simulink model "dac_driver"  (R2012b)
settings: Solver=ode45  StartTime=0.0  StopTime=10.0  RelTol=1e-3
undefined symbols (not defined in the file or in its folder): gcbh, xlBlockLoadCallback, xlGetNormalizedPeriod
libraries: xbsIndex_r4 x54, xbsEDKLib_r4 x1
(part 1 of 2)
settings Model: Creator=rcagley  LastModifiedBy=rcagley
settings DataIOCC: SignalLoggingSaveFormat=ModelDataLogs
settings DebuggingCC: FcnCallInpInsideContextMsg=EnableAllAsWarning

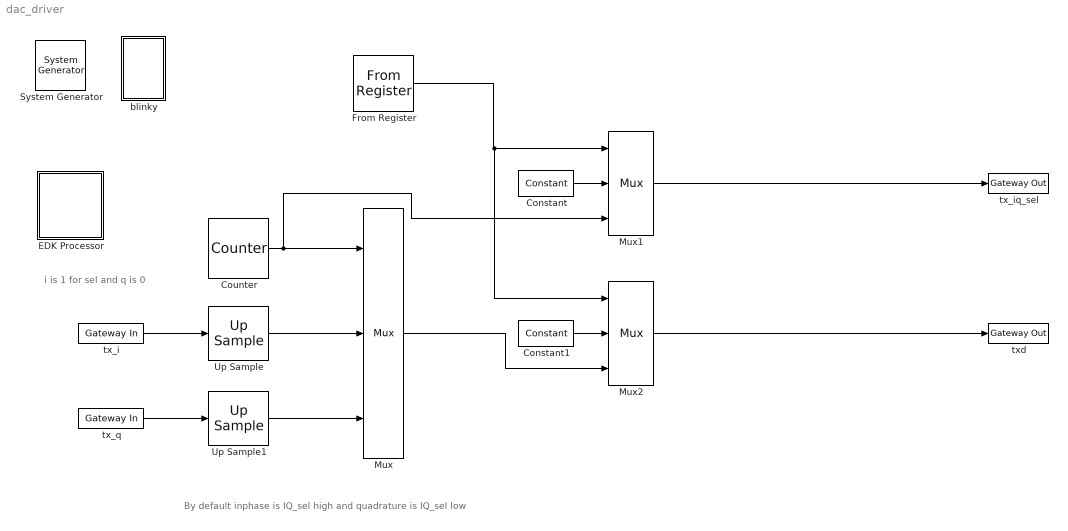
== system dac_driver ==
  note: i is 1 for sel and q is 0
  note: By default inphase is IQ_sel high and quadrature is IQ_sel low
  " System Generator" : xbsIndex_r4/ System Generator  Tag=genX  xilinxfamily=zynq  part=xc7z020  speed=-1  package=clg484  synthesis_tool=XST  clock_wrapper=Clock Enables  directory=./netlist  proj_type=Project Navigator  Synth_file=XST Defaults  Impl_file=ISE Defaults  testbench=off  simulink_period=1  sysclk_period=10  dcm_input_clock_period=10  incr_netlist=off  trim_vbits=Everywhere in SubSystem  dbl_ovrd=According to Block Masks  core_generation=According to Block Masks  run_coregen=off  deprecated_control=off  eval_field=0  block_type=sysgen
  Constant : xbsIndex_r4/Constant  const=0  gui_display_data_type=Fixed-point  arith_type=Unsigned  n_bits=1  bin_pt=0  preci_type=Single  exp_width=8  frac_width=24  explicit_period=on  period=1  equ=P=C  opselect=C  inp2=PCIN>>17  opr=+  inp1=P  carry=CIN  dbl_ovrd=off  block_type=constant
  Constant1 : xbsIndex_r4/Constant  const=0  gui_display_data_type=Fixed-point  arith_type=Signed (2's comp)  n_bits=12  bin_pt=0  preci_type=Single  exp_width=8  frac_width=24  explicit_period=on  period=1  equ=P=C  opselect=C  inp2=PCIN>>17  opr=+  inp1=P  carry=CIN  dbl_ovrd=off  block_type=constant
  Counter : xbsIndex_r4/Counter  cnt_type=Free Running  cnt_to=Inf  operation=Up  start_count=0  cnt_by_val=1  arith_type=Unsigned  n_bits=1  bin_pt=0  load_pin=off  rst=off  en=off  explicit_period=on  period=1  dbl_ovrd=off  use_behavioral_HDL=off  implementation=Fabric  block_type=counter
  EDK Processor : Subsystem  LoadFcn=xlBlockLoadCallback(gcbh);  mask(Xilinx EDK Processor Block){mode=EDK pcore generation, xmp=, MemVisToProc=<qt bgcolor="#FFFFFF"><div><img src="C:/Xilinx/14.2/ISE_DS/ISE/sysgen/data/images/registerplus.gif"> &lt;&lt;dac_en&gt;&gt;<br></div></qt>, AvailableMemories=<empty>, portInterfaceTable={'exposed'=>[],'portdir'=>[],'portname'=>[],'shortname'=>[]}, bus_type_sgadvanced=, bus_type=AXI, baseaddr=0x80000000, baseaddr_lock_sgadvanced=, baseaddr_lock=off, dual_clock_sgadvanced=, dual_clock=on, reg_readback_sgadvanced=, reg_readback=off, ucf_file=, inheritDeviceType_sgadvanced=, inheritDeviceType=off, elf_file=, codebug_sgadvanced=, codebug=on, clock_name=plb, internalPortList={}, resetPolarity=0, memxtable={'mladdr'=>[0.00000000000000000],'mlist'=>['dac_driver/From Register'],'mlname'=>['\'dac_en\''],'mlstate'=>[0.00000000000000000]}, procinfo={}, memmapdirty=off, blockname=, xpsintstyle=default, has_advanced_control=0, sggui_pos=-1,-1,-1,-1, block_type=edkprocessor, block_version=2.7, sg_icon_stat=62,64,-1,-1,white,blue,0,07734,right,,[ ],[ ], sg_mask_display=|, sg_list_contents={'table'=>{'AvailableMemories'=>'popup(<empty>)'}}, sg_blockgui_xml=}
      mask sg_mask_display=|
      | fprintf('','COMMENT: begin icon graphics');
      | patch([0 62 62 0 0 ],[0 0 64 64 0 ],[0.77 0.82 0.91 ]);
      | plot([0 62 62 0 0 ],[0 0 64 64 0 ]);
      | patch([13.2 24.76 32.76 40.76 48.76 32.76 21.2 13.2 ],[40.88 40.88 48.88 40.88 48.88 48.88 48.88 40.88 ],[1 1 1 ]);
      | patch([21.2 32.76 24.76 13.2 21.2 ],[32.88 32.88 40.88 40.88 32.88 ],[0.931 0.946 0.973 ]);
      | patch([13.2 24.76 32.76 21.2 13.2 ],[24.88 24.88 32.88 32.88 24.88 ],[1 1 1 ]);
      | patch([21.2 48.76 40.76 32.76 24.76 13.2 21.2 ],[16.88 16.88 24.88 16.88 24.88 24.88 16.88 ],[0.931 0.946 0.973 ]);
      | fprintf('','COMMENT: end icon graphics');
      | fprintf('','COMMENT: begin icon text');
      | fprintf('','COMMENT: end icon text');
      mask prompts: mode "Configure Processor for"; xmp "XPS Project"; MemVisToProc ""; AvailableMemories "Available Memories"; portInterfaceTable ""; bus_type_sgadvanced ""; bus_type "Bus Type"; baseaddr "Base Address"; baseaddr_lock_sgadvanced ""; baseaddr_lock "Lock"; dual_clock_sgadvanced ""; dual_clock "Dual Clocks"; reg_readback_sgadvanced ""; reg_readback "Register Read-Back"; ucf_file "Constraint File"; inheritDeviceType_sgadvanced ""; inheritDeviceType "Inherit Device Type"; elf_file "Initial Program"; codebug_sgadvanced ""; codebug "Enable Co-Debug with Xilinx SDK (Beta)"; clock_name ""; internalPortList ""; resetPolarity ""; memxtable ""; procinfo ""; memmapdirty ""; blockname ""; xpsintstyle ""; has_advanced_control ""; sggui_pos ""; block_type ""; block_version ""; sg_icon_stat ""; sg_mask_display ""; sg_list_contents ""; sg_blockgui_xml ""
      mask help: Xilinx EDK Processor
      mask init:
      | try
      |   tmp_gcb = gcb;
      |   tmp_gcbh = gcbh;
      |   if (strcmp('SysGenIndex',get_param(bdroot(tmp_gcbh),'tag')) && ~isempty(regexp(bdroot(tmp_gcb), '^xbs', 'once')))
      |     return;
      |   end;
      |   xlMungeMaskParams;
      | 
      |   block_type='edkprocessor';
      | 
      |   serialized_declarations = '{''block_type''=>''String''}';
      |   xledkprocessor_init();
      |   ptable_ = xlblockprep(get_param(tmp_gcb, 'MaskWSVariables'));
      |   try
      |     xlBlockMoveCallback(tmp_gcbh);
      |   catch 
      |      clear global xl_updateicon_recursion_guard;
      |   end;
      | catch
      |   global dbgsysgen;
      |   if(~isempty(dbgsysgen) && dbgsysgen)
      |     e = regexprep(lasterr, '\n', '\nError: ');
      |     disp(['Error: While running MaskInit code on block ' tmp_gcb ': ' e]);
      |     error(e);
      |   end
      | end
      settings: CopyFcn=xlProcBlockCopyCallback(gcbh);xlBlockMoveCallback(gcbh);  DeleteFcn=xlDestroyGui(gcbh);  ModelCloseFcn=xlDestroyGui(gcbh);  PreSaveFcn=xlBlockPreSaveCallback(gcbh);  PostSaveFcn=xlBlockPostSaveCallback(gcbh);  DestroyFcn=xlDestroyGui(gcbh);  OpenFcn=bh=gcbh;xlProcBlockCallbacks('populatesharedmemorylistbox',bh);xlOpenGui(bh, 'edkprocessor_gui.xml', @xlProcBlockEnablement, @xlProcBlockAction);  CloseFcn=xlDestroyGui(gcbh);  MoveFcn=xlBlockMoveCallback(gcbh);
      mask Help: eval('');xlDoc('-book','sysgen','-topic','EDK_Processor');
      mask TypeOptions mode: EDK pcore generation | HDL netlisting
      mask TypeOptions bus_type: AXI | PLB
      mask Display:
      | fprintf('','COMMENT: begin icon graphics');
      | patch([0 62 62 0 0 ],[0 0 64 64 0 ],[0.77 0.82 0.91 ]);
      | plot([0 62 62 0 0 ],[0 0 64 64 0 ]);
      | patch([13.2 24.76 32.76 40.76 48.76 32.76 21.2 13.2 ],[40.88 40.88 48.88 40.88 48.88 48.88 48.88 40.88 ],[1 1 1 ]);
      | patch([21.2 32.76 24.76 13.2 21.2 ],[32.88 32.88 40.88 40.88 32.88 ],[0.931 0.946 0.973 ]);
      | patch([13.2 24.76 32.76 21.2 13.2 ],[24.88 24.88 32.88 32.88 24.88 ],[1 1 1 ]);
      | patch([21.2 48.76 40.76 32.76 24.76 13.2 21.2 ],[16.88 16.88 24.88 16.88 24.88 24.88 16.88 ],[0.931 0.946 0.973 ]);
      | fprintf('','COMMENT: end icon graphics');
      | fprintf('','COMMENT: begin icon text');
      | disp('');
      | 
      | fprintf('','COMMENT: end icon text');
  From Register : xbsIndex_r4/From Register  shared_memory_name='dac_en'  init=0  period=1  ownership=Locally owned and initialized  gui_display_data_type=Fixed-point  arith_type=Unsigned  n_bits=1  bin_pt=0  preci_type=Single  dbl_ovrd=off  block_type=fromreg
      settings: AttributesFormatString=<< %<shared_memory_name> >>  infoedit="Register block that reads data to a shared memory register.  Delay of one sample period."
  Mux : xbsIndex_r4/Mux  inputs=2  en=off  latency=0  precision=Full  arith_type=Unsigned  n_bits=16  bin_pt=14  quantization=Truncate  overflow=Wrap  dbl_ovrd=off  block_type=mux
  Mux1 : xbsIndex_r4/Mux  inputs=2  en=off  latency=0  precision=Full  arith_type=Unsigned  n_bits=16  bin_pt=14  quantization=Truncate  overflow=Wrap  dbl_ovrd=off  block_type=mux
  Mux2 : xbsIndex_r4/Mux  inputs=2  en=off  latency=0  precision=Full  arith_type=Unsigned  n_bits=16  bin_pt=14  quantization=Truncate  overflow=Wrap  dbl_ovrd=off  block_type=mux
  Up Sample : xbsIndex_r4/Up Sample  sample_ratio=2  copy_samples=on  en=off  latency=0  dbl_ovrd=off  block_type=usamp
  Up Sample1 : xbsIndex_r4/Up Sample  sample_ratio=2  copy_samples=on  en=off  latency=0  dbl_ovrd=off  block_type=usamp
  blinky : Subsystem
  tx_i : xbsIndex_r4/Gateway In  gui_display_data_type=Fixed-point  arith_type="Signed  (2's comp)"  n_bits=12  bin_pt=0  preci_type=Single  exp_width=8  frac_width=24  quantization="Round  (unbiased: +/- Inf)"  overflow=Saturate  period=2  dbl_ovrd=off  timing_constraint=None  locs_specified=off  LOCs={}  UseAsADC=off  ADCChannel='1'  inherit_from_input=off  hdl_port=on  block_type=gatewayin
  tx_iq_sel : xbsIndex_r4/Gateway Out  inherit_from_input=off  hdl_port=on  timing_constraint=None  locs_specified=off  LOCs={}  UseAsDAC=off  DACChannel='1'  block_type=gatewayout
  tx_q : xbsIndex_r4/Gateway In  gui_display_data_type=Fixed-point  arith_type="Signed  (2's comp)"  n_bits=12  bin_pt=0  preci_type=Single  exp_width=8  frac_width=24  quantization="Round  (unbiased: +/- Inf)"  overflow=Saturate  period=2  dbl_ovrd=off  timing_constraint=None  locs_specified=off  LOCs={}  UseAsADC=off  ADCChannel='1'  inherit_from_input=off  hdl_port=on  block_type=gatewayin
  txd : xbsIndex_r4/Gateway Out  inherit_from_input=off  hdl_port=on  timing_constraint=None  locs_specified=off  LOCs={}  UseAsDAC=off  DACChannel='1'  block_type=gatewayout
  wires:
  Up Sample/1 -> Mux/2
  Up Sample1/1 -> Mux/3
  Counter/1 -> Mux/1, Mux1/3
  Mux2/1 -> txd/1
  Mux1/1 -> tx_iq_sel/1
  Mux/1 -> Mux2/3
  From Register/1 -> Mux2/1, Mux1/1
  Constant/1 -> Mux1/2
  Constant1/1 -> Mux2/2
  tx_i/1 -> Up Sample/1
  tx_q/1 -> Up Sample1/1

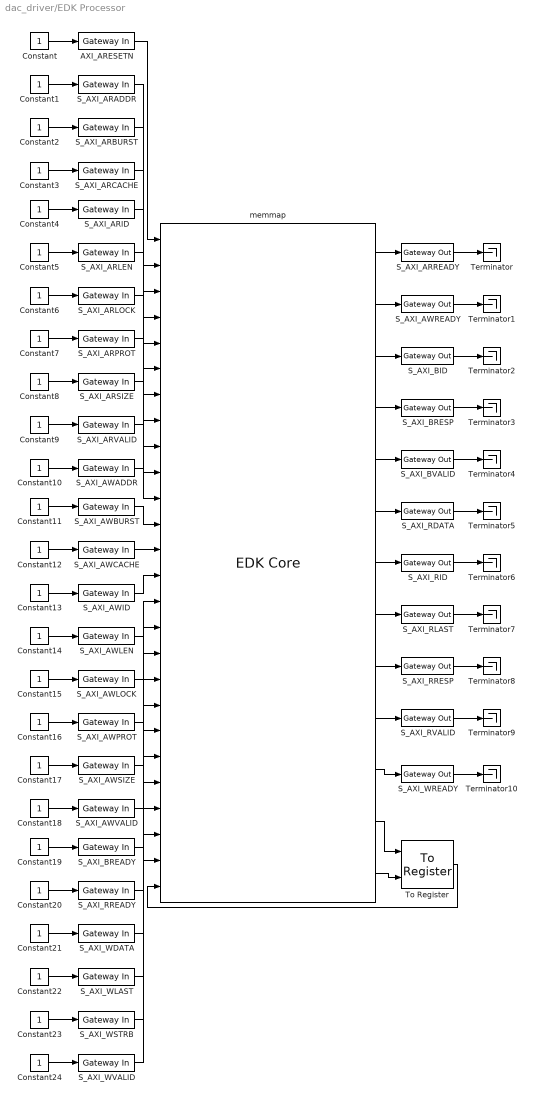
== system dac_driver/EDK Processor ==
  AXI_ARESETN : xbsIndex_r4/Gateway In  gui_display_data_type=Fixed-point  arith_type=Boolean  n_bits=16  bin_pt=14  preci_type=Single  exp_width=8  frac_width=24  quantization="Round  (unbiased: +/- Inf)"  overflow=Saturate  period=xlGetNormalizedPeriod()  dbl_ovrd=off  timing_constraint=None  locs_specified=off  LOCs={}  UseAsADC=off  ADCChannel='1'  inherit_from_input=off  hdl_port=on  block_type=gatewayin
  Constant{,1..24} (25 alike) : Constant
  S_AXI_ARADDR : xbsIndex_r4/Gateway In  gui_display_data_type=Fixed-point  arith_type=Unsigned  n_bits=32  bin_pt=0  preci_type=Single  exp_width=8  frac_width=24  quantization="Round  (unbiased: +/- Inf)"  overflow=Saturate  period=xlGetNormalizedPeriod()  dbl_ovrd=off  timing_constraint=None  locs_specified=off  LOCs={}  UseAsADC=off  ADCChannel='1'  inherit_from_input=off  hdl_port=on  block_type=gatewayin
  S_AXI_ARBURST : xbsIndex_r4/Gateway In  gui_display_data_type=Fixed-point  arith_type=Unsigned  n_bits=2  bin_pt=0  preci_type=Single  exp_width=8  frac_width=24  quantization="Round  (unbiased: +/- Inf)"  overflow=Saturate  period=xlGetNormalizedPeriod()  dbl_ovrd=off  timing_constraint=None  locs_specified=off  LOCs={}  UseAsADC=off  ADCChannel='1'  inherit_from_input=off  hdl_port=on  block_type=gatewayin
  S_AXI_ARCACHE : xbsIndex_r4/Gateway In  gui_display_data_type=Fixed-point  arith_type=Unsigned  n_bits=4  bin_pt=0  preci_type=Single  exp_width=8  frac_width=24  quantization="Round  (unbiased: +/- Inf)"  overflow=Saturate  period=xlGetNormalizedPeriod()  dbl_ovrd=off  timing_constraint=None  locs_specified=off  LOCs={}  UseAsADC=off  ADCChannel='1'  inherit_from_input=off  hdl_port=on  block_type=gatewayin
  S_AXI_ARID : xbsIndex_r4/Gateway In  gui_display_data_type=Fixed-point  arith_type=Unsigned  n_bits=8  bin_pt=0  preci_type=Single  exp_width=8  frac_width=24  quantization="Round  (unbiased: +/- Inf)"  overflow=Saturate  period=xlGetNormalizedPeriod()  dbl_ovrd=off  timing_constraint=None  locs_specified=off  LOCs={}  UseAsADC=off  ADCChannel='1'  inherit_from_input=off  hdl_port=on  block_type=gatewayin
  S_AXI_ARLEN : xbsIndex_r4/Gateway In  gui_display_data_type=Fixed-point  arith_type=Unsigned  n_bits=8  bin_pt=0  preci_type=Single  exp_width=8  frac_width=24  quantization="Round  (unbiased: +/- Inf)"  overflow=Saturate  period=xlGetNormalizedPeriod()  dbl_ovrd=off  timing_constraint=None  locs_specified=off  LOCs={}  UseAsADC=off  ADCChannel='1'  inherit_from_input=off  hdl_port=on  block_type=gatewayin
  S_AXI_ARLOCK : xbsIndex_r4/Gateway In  gui_display_data_type=Fixed-point  arith_type=Unsigned  n_bits=2  bin_pt=0  preci_type=Single  exp_width=8  frac_width=24  quantization="Round  (unbiased: +/- Inf)"  overflow=Saturate  period=xlGetNormalizedPeriod()  dbl_ovrd=off  timing_constraint=None  locs_specified=off  LOCs={}  UseAsADC=off  ADCChannel='1'  inherit_from_input=off  hdl_port=on  block_type=gatewayin
  S_AXI_ARPROT : xbsIndex_r4/Gateway In  gui_display_data_type=Fixed-point  arith_type=Unsigned  n_bits=3  bin_pt=0  preci_type=Single  exp_width=8  frac_width=24  quantization="Round  (unbiased: +/- Inf)"  overflow=Saturate  period=xlGetNormalizedPeriod()  dbl_ovrd=off  timing_constraint=None  locs_specified=off  LOCs={}  UseAsADC=off  ADCChannel='1'  inherit_from_input=off  hdl_port=on  block_type=gatewayin
  S_AXI_ARREADY : xbsIndex_r4/Gateway Out  inherit_from_input=off  hdl_port=on  timing_constraint=None  locs_specified=off  LOCs={}  UseAsDAC=off  DACChannel='1'  block_type=gatewayout
  S_AXI_ARSIZE : xbsIndex_r4/Gateway In  gui_display_data_type=Fixed-point  arith_type=Unsigned  n_bits=3  bin_pt=0  preci_type=Single  exp_width=8  frac_width=24  quantization="Round  (unbiased: +/- Inf)"  overflow=Saturate  period=xlGetNormalizedPeriod()  dbl_ovrd=off  timing_constraint=None  locs_specified=off  LOCs={}  UseAsADC=off  ADCChannel='1'  inherit_from_input=off  hdl_port=on  block_type=gatewayin
  S_AXI_ARVALID : xbsIndex_r4/Gateway In  gui_display_data_type=Fixed-point  arith_type=Boolean  n_bits=16  bin_pt=14  preci_type=Single  exp_width=8  frac_width=24  quantization="Round  (unbiased: +/- Inf)"  overflow=Saturate  period=xlGetNormalizedPeriod()  dbl_ovrd=off  timing_constraint=None  locs_specified=off  LOCs={}  UseAsADC=off  ADCChannel='1'  inherit_from_input=off  hdl_port=on  block_type=gatewayin
  S_AXI_AWADDR : xbsIndex_r4/Gateway In  gui_display_data_type=Fixed-point  arith_type=Unsigned  n_bits=32  bin_pt=0  preci_type=Single  exp_width=8  frac_width=24  quantization="Round  (unbiased: +/- Inf)"  overflow=Saturate  period=xlGetNormalizedPeriod()  dbl_ovrd=off  timing_constraint=None  locs_specified=off  LOCs={}  UseAsADC=off  ADCChannel='1'  inherit_from_input=off  hdl_port=on  block_type=gatewayin
  S_AXI_AWBURST : xbsIndex_r4/Gateway In  gui_display_data_type=Fixed-point  arith_type=Unsigned  n_bits=2  bin_pt=0  preci_type=Single  exp_width=8  frac_width=24  quantization="Round  (unbiased: +/- Inf)"  overflow=Saturate  period=xlGetNormalizedPeriod()  dbl_ovrd=off  timing_constraint=None  locs_specified=off  LOCs={}  UseAsADC=off  ADCChannel='1'  inherit_from_input=off  hdl_port=on  block_type=gatewayin
  S_AXI_AWCACHE : xbsIndex_r4/Gateway In  gui_display_data_type=Fixed-point  arith_type=Unsigned  n_bits=4  bin_pt=0  preci_type=Single  exp_width=8  frac_width=24  quantization="Round  (unbiased: +/- Inf)"  overflow=Saturate  period=xlGetNormalizedPeriod()  dbl_ovrd=off  timing_constraint=None  locs_specified=off  LOCs={}  UseAsADC=off  ADCChannel='1'  inherit_from_input=off  hdl_port=on  block_type=gatewayin
  S_AXI_AWID : xbsIndex_r4/Gateway In  gui_display_data_type=Fixed-point  arith_type=Unsigned  n_bits=8  bin_pt=0  preci_type=Single  exp_width=8  frac_width=24  quantization="Round  (unbiased: +/- Inf)"  overflow=Saturate  period=xlGetNormalizedPeriod()  dbl_ovrd=off  timing_constraint=None  locs_specified=off  LOCs={}  UseAsADC=off  ADCChannel='1'  inherit_from_input=off  hdl_port=on  block_type=gatewayin
  S_AXI_AWLEN : xbsIndex_r4/Gateway In  gui_display_data_type=Fixed-point  arith_type=Unsigned  n_bits=8  bin_pt=0  preci_type=Single  exp_width=8  frac_width=24  quantization="Round  (unbiased: +/- Inf)"  overflow=Saturate  period=xlGetNormalizedPeriod()  dbl_ovrd=off  timing_constraint=None  locs_specified=off  LOCs={}  UseAsADC=off  ADCChannel='1'  inherit_from_input=off  hdl_port=on  block_type=gatewayin
  S_AXI_AWLOCK : xbsIndex_r4/Gateway In  gui_display_data_type=Fixed-point  arith_type=Unsigned  n_bits=2  bin_pt=0  preci_type=Single  exp_width=8  frac_width=24  quantization="Round  (unbiased: +/- Inf)"  overflow=Saturate  period=xlGetNormalizedPeriod()  dbl_ovrd=off  timing_constraint=None  locs_specified=off  LOCs={}  UseAsADC=off  ADCChannel='1'  inherit_from_input=off  hdl_port=on  block_type=gatewayin
  S_AXI_AWPROT : xbsIndex_r4/Gateway In  gui_display_data_type=Fixed-point  arith_type=Unsigned  n_bits=3  bin_pt=0  preci_type=Single  exp_width=8  frac_width=24  quantization="Round  (unbiased: +/- Inf)"  overflow=Saturate  period=xlGetNormalizedPeriod()  dbl_ovrd=off  timing_constraint=None  locs_specified=off  LOCs={}  UseAsADC=off  ADCChannel='1'  inherit_from_input=off  hdl_port=on  block_type=gatewayin
  S_AXI_AWREADY : xbsIndex_r4/Gateway Out  inherit_from_input=off  hdl_port=on  timing_constraint=None  locs_specified=off  LOCs={}  UseAsDAC=off  DACChannel='1'  block_type=gatewayout
  S_AXI_AWSIZE : xbsIndex_r4/Gateway In  gui_display_data_type=Fixed-point  arith_type=Unsigned  n_bits=3  bin_pt=0  preci_type=Single  exp_width=8  frac_width=24  quantization="Round  (unbiased: +/- Inf)"  overflow=Saturate  period=xlGetNormalizedPeriod()  dbl_ovrd=off  timing_constraint=None  locs_specified=off  LOCs={}  UseAsADC=off  ADCChannel='1'  inherit_from_input=off  hdl_port=on  block_type=gatewayin
  S_AXI_AWVALID : xbsIndex_r4/Gateway In  gui_display_data_type=Fixed-point  arith_type=Boolean  n_bits=16  bin_pt=14  preci_type=Single  exp_width=8  frac_width=24  quantization="Round  (unbiased: +/- Inf)"  overflow=Saturate  period=xlGetNormalizedPeriod()  dbl_ovrd=off  timing_constraint=None  locs_specified=off  LOCs={}  UseAsADC=off  ADCChannel='1'  inherit_from_input=off  hdl_port=on  block_type=gatewayin
  S_AXI_BID : xbsIndex_r4/Gateway Out  inherit_from_input=off  hdl_port=on  timing_constraint=None  locs_specified=off  LOCs={}  UseAsDAC=off  DACChannel='1'  block_type=gatewayout
  S_AXI_BREADY : xbsIndex_r4/Gateway In  gui_display_data_type=Fixed-point  arith_type=Boolean  n_bits=16  bin_pt=14  preci_type=Single  exp_width=8  frac_width=24  quantization="Round  (unbiased: +/- Inf)"  overflow=Saturate  period=xlGetNormalizedPeriod()  dbl_ovrd=off  timing_constraint=None  locs_specified=off  LOCs={}  UseAsADC=off  ADCChannel='1'  inherit_from_input=off  hdl_port=on  block_type=gatewayin
  S_AXI_BRESP : xbsIndex_r4/Gateway Out  inherit_from_input=off  hdl_port=on  timing_constraint=None  locs_specified=off  LOCs={}  UseAsDAC=off  DACChannel='1'  block_type=gatewayout
  S_AXI_BVALID : xbsIndex_r4/Gateway Out  inherit_from_input=off  hdl_port=on  timing_constraint=None  locs_specified=off  LOCs={}  UseAsDAC=off  DACChannel='1'  block_type=gatewayout
  S_AXI_RDATA : xbsIndex_r4/Gateway Out  inherit_from_input=off  hdl_port=on  timing_constraint=None  locs_specified=off  LOCs={}  UseAsDAC=off  DACChannel='1'  block_type=gatewayout
  S_AXI_RID : xbsIndex_r4/Gateway Out  inherit_from_input=off  hdl_port=on  timing_constraint=None  locs_specified=off  LOCs={}  UseAsDAC=off  DACChannel='1'  block_type=gatewayout
  S_AXI_RLAST : xbsIndex_r4/Gateway Out  inherit_from_input=off  hdl_port=on  timing_constraint=None  locs_specified=off  LOCs={}  UseAsDAC=off  DACChannel='1'  block_type=gatewayout
  S_AXI_RREADY : xbsIndex_r4/Gateway In  gui_display_data_type=Fixed-point  arith_type=Boolean  n_bits=16  bin_pt=14  preci_type=Single  exp_width=8  frac_width=24  quantization="Round  (unbiased: +/- Inf)"  overflow=Saturate  period=xlGetNormalizedPeriod()  dbl_ovrd=off  timing_constraint=None  locs_specified=off  LOCs={}  UseAsADC=off  ADCChannel='1'  inherit_from_input=off  hdl_port=on  block_type=gatewayin
  S_AXI_RRESP : xbsIndex_r4/Gateway Out  inherit_from_input=off  hdl_port=on  timing_constraint=None  locs_specified=off  LOCs={}  UseAsDAC=off  DACChannel='1'  block_type=gatewayout
  S_AXI_RVALID : xbsIndex_r4/Gateway Out  inherit_from_input=off  hdl_port=on  timing_constraint=None  locs_specified=off  LOCs={}  UseAsDAC=off  DACChannel='1'  block_type=gatewayout
  S_AXI_WDATA : xbsIndex_r4/Gateway In  gui_display_data_type=Fixed-point  arith_type=Unsigned  n_bits=32  bin_pt=0  preci_type=Single  exp_width=8  frac_width=24  quantization="Round  (unbiased: +/- Inf)"  overflow=Saturate  period=xlGetNormalizedPeriod()  dbl_ovrd=off  timing_constraint=None  locs_specified=off  LOCs={}  UseAsADC=off  ADCChannel='1'  inherit_from_input=off  hdl_port=on  block_type=gatewayin
  S_AXI_WLAST : xbsIndex_r4/Gateway In  gui_display_data_type=Fixed-point  arith_type=Boolean  n_bits=16  bin_pt=14  preci_type=Single  exp_width=8  frac_width=24  quantization="Round  (unbiased: +/- Inf)"  overflow=Saturate  period=xlGetNormalizedPeriod()  dbl_ovrd=off  timing_constraint=None  locs_specified=off  LOCs={}  UseAsADC=off  ADCChannel='1'  inherit_from_input=off  hdl_port=on  block_type=gatewayin
  S_AXI_WREADY : xbsIndex_r4/Gateway Out  inherit_from_input=off  hdl_port=on  timing_constraint=None  locs_specified=off  LOCs={}  UseAsDAC=off  DACChannel='1'  block_type=gatewayout
  S_AXI_WSTRB : xbsIndex_r4/Gateway In  gui_display_data_type=Fixed-point  arith_type=Unsigned  n_bits=4  bin_pt=0  preci_type=Single  exp_width=8  frac_width=24  quantization="Round  (unbiased: +/- Inf)"  overflow=Saturate  period=xlGetNormalizedPeriod()  dbl_ovrd=off  timing_constraint=None  locs_specified=off  LOCs={}  UseAsADC=off  ADCChannel='1'  inherit_from_input=off  hdl_port=on  block_type=gatewayin
  S_AXI_WVALID : xbsIndex_r4/Gateway In  gui_display_data_type=Fixed-point  arith_type=Boolean  n_bits=16  bin_pt=14  preci_type=Single  exp_width=8  frac_width=24  quantization="Round  (unbiased: +/- Inf)"  overflow=Saturate  period=xlGetNormalizedPeriod()  dbl_ovrd=off  timing_constraint=None  locs_specified=off  LOCs={}  UseAsADC=off  ADCChannel='1'  inherit_from_input=off  hdl_port=on  block_type=gatewayin
  Terminator{,1..10} (11 alike) : Terminator
  To Register : xbsIndex_r4/To Register  shared_memory_name='dac_en'  init=0  ownership=Owned and initialized elsewhere  explicit_data_type=on  gui_display_data_type=Fixed-point  arith_type=Unsigned  n_bits=1  bin_pt=0  preci_type=Single  dbl_ovrd=off  block_type=toreg
      settings: AttributesFormatString=<< %<shared_memory_name> >>  infoedit="Register block that writes data to a shared memory register.  Delay of one sample period."
  memmap : xbsEDKLib_r4/EDK Core  sim_method=Inactive  xmp=xmp  blockname=blockname  dual_clock=dual_clock  procinfo=procinfo  bus_type=bus_type  memxtable=memxtable  memmap_hdlcontent=|  config={'inports'=>[{'arith_type'=>2.00000000000000000,'bin_pt'=>0.00000000000000000,'name'=>'AXI_ARESETN','width'=>0},{'arith_type'=>2.00000000000000000,'bin_pt'=>0.00000000000000000,'name'=>'S_AXI_ARADDR','width'=>32},{'arith_type'=>2.00000000000000000,'bin_pt'=>0.00000000000000000,'name'=>'S_AXI_ARBURST','width'=>2},{'arith_type'=>2.00000000000000000,'bin_pt'=>0.00000000000000000,'name'=>'S_AXI_ARCACHE','width'=>4},{'arith_type'=>2.00000000000000000,'bin_pt'=>0.00000000000000000,'name'=>'S_AXI_ARID','width'=>8},{'arith_type'=>2.00000000000000000,'bin_pt'=>0.00000000000000000,'name'=>'S_AXI_ARLEN','width'=>8},{'arith_type'=>2.00000000000000000,'bin_pt'=>0.00000000000000000,'name'=>'S_AXI_ARLOCK','width'=>2},{'arith_type'=>2.00000000000000000,'bin_pt'=>0.00000000000000000,'name'=>'S_AXI_ARPROT','width'=>3},{'arith_type'=>2.00000000000000000,'bin_pt'=>0.00000000000000000,'name'=>'S_AXI_ARSIZE','width'=>3},{'arith_type'=>2.00000000000000000,'bin_pt'=>0.00000000000000000,'name'=>'S_AXI_ARVALID','width'=>0},{'arith_type'=>2.00000000000000000,'bin_pt'=>0.00000000000000000,'name'=>'S_AXI_AWADDR','width'=>32},{'arith_type'=>2.00000000000000000,'bin_pt'=>0.00000000000000000,'name'=>'S_AXI_AWBURST','width'=>2},{'arith_type'=>2.00000000000000000,'bin_pt'=>0.00000000000000000,'name'=>'S_AXI_AWCACHE','width'=>4},{'arith_type'=>2.00000000000000000,'bin_pt'=>0.00000000000000000,'name'=>'S_AXI_AWID','width'=>8},{'arith_type'=>2.00000000000000000,'bin_pt'=>0.00000000000000000,'name'=>'S_AXI_AWLEN','width'=>8},{'arith_type'=>2.00000000000000000,'bin_pt'=>0.00000000000000000,'name'=>'S_AXI_AWLOCK','width'=>2},{'arith_type'=>2.00000000000000000,'bin_pt'=>0.00000000000000000,'name'=>'S_AXI_AWPROT','width'=>3},{'arith_type'=>2.00000000000000000,'bin_pt'=>0.00000000000000000,'name'=>'S_AXI_AWSIZE','width'=>3},{'arith_type'=>2.00000000000000000,'bin_pt'=>0.00000000000000000,'name'=>'S_AXI_AWVALID','width'=>0},{'arith_type'=>2.00000000000000000,'bin_pt'=>0.00000000000000000,'name'=>'S_AXI_BREADY','width'=>0},{'arith_type'=>2.00000000000000000,'bin_pt'=>0.00000000000000000,'name'=>'S_AXI_RREADY','width'=>0},{'arith_type'=>2.00000000000000000,'bin_pt'=>0.00000000000000000,'name'=>'S_AXI_WDATA','width'=>32},{'arith_type'=>2.00000000000000000,'bin_pt'=>0.00000000000000000,'name'=>'S_AXI_WLAST','width'=>0},{'arith_type'=>2.00000000000000000,'bin_pt'=>0.00000000000000000,'name'=>'S_AXI_WSTRB','width'=>4},{'arith_type'=>2.00000000000000000,'bin_pt'=>0.00000000000000000,'name'=>'S_AXI_WVALID','width'=>0},{'arith_type'=>2,'bin_pt'=>0,'name'=>'sm_dac_en_dout','width'=>1}],'outports'=>[{'arith_type'=>2.00000000000000000,'bin_pt'=>0.00000000000000000,'name'=>'S_AXI_ARREADY','width'=>0},{'arith_type'=>2.00000000000000000,'bin_pt'=>0.00000000000000000,'name'=>'S_AXI_AWREADY','width'=>0},{'arith_type'=>2.00000000000000000,'bin_pt'=>0.00000000000000000,'name'=>'S_AXI_BID','width'=>8},{'arith_type'=>2.00000000000000000,'bin_pt'=>0.00000000000000000,'name'=>'S_AXI_BRESP','width'=>2},{'arith_type'=>2.00000000000000000,'bin_pt'=>0.00000000000000000,'name'=>'S_AXI_BVALID','width'=>0},{'arith_type'=>2.00000000000000000,'bin_pt'=>0.00000000000000000,'name'=>'S_AXI_RDATA','width'=>32},{'arith_type'=>2.00000000000000000,'bin_pt'=>0.00000000000000000,'name'=>'S_AXI_RID','width'=>8},{'arith_type'=>2.00000000000000000,'bin_pt'=>0.00000000000000000,'name'=>'S_AXI_RLAST','width'=>0},{'arith_type'=>2.00000000000000000,'bin_pt'=>0.00000000000000000,'name'=>'S_AXI_RRESP','width'=>2},{'arith_type'=>2.00000000000000000,'bin_pt'=>0.00000000000000000,'name'=>'S_AXI_RVALID','width'=>0},{'arith_type'=>2.00000000000000000,'bin_pt'=>0.00000000000000000,'name'=>'S_AXI_WREADY','width'=>0},{'arith_type'=>2,'bin_pt'=>0,'name'=>'sm_dac_en_din','width'=>1},{'arith_type'=>2.00000000000000000,'bin_pt'=>0.00000000000000000,'name'=>'sm_dac_en_en','width'=>0.00000000000000000}]}  inheritDeviceType=inheritDeviceType  block_type=edkcore
      | library IEEE;
      | use IEEE.std_logic_1164.all;
      | use IEEE.numeric_std.all;
      | 
      | entity axi_sgiface is
      |     generic (
      |         -- AXI specific.
      |         -- TODO: need to figure out a way to pass these generics from outside
      |         C_S_AXI_SUPPORT_BURST   : integer := 0;
      |         -- TODO: fix the internal ID width to 8
      |         C_S_AXI_ID_WIDTH        : integer := 8;
      |         C_S_AXI_DATA_WIDTH      : integer := 32;
      |         C_S_AXI_ADDR_WIDTH      : integer := 32;
      |         C_S_AXI_TOTAL_ADDR_LEN  : integer := 12;
      |         C_S_AXI_LINEAR_ADDR_LEN : integer := 8;
      |         C_S_AXI_BANK_ADDR_LEN   : integer := 2;
      |         C_S_AXI_AWLEN_WIDTH     : integer := 8;
      |         C_S_AXI_ARLEN_WIDTH     : integer := 8
      |     );
      |     port (
      |         -- General.
      |         AXI_AClk      : in  std_logic;
      |         AXI_AResetN    : in  std_logic;
      |         -- not used
      |         AXI_Ce        : in  std_logic;
      |   
      |         -- AXI Port.
      |         S_AXI_AWADDR  : in  std_logic_vector(C_S_AXI_ADDR_WIDTH-1 downto 0);
      |         S_AXI_AWID    : in  std_logic_vector(C_S_AXI_ID_WIDTH-1 downto 0);
      |         S_AXI_AWLEN   : in  std_logic_vector(C_S_AXI_AWLEN_WIDTH-1 downto 0);
      |         S_AXI_AWSIZE  : in  std_logic_vector(2 downto 0);
      |         S_AXI_AWBURST : in  std_logic_vector(1 downto 0);
      |         S_AXI_AWLOCK  : in  std_logic_vector(1 downto 0);
      |         S_AXI_AWCACHE : in  std_logic_vector(3 downto 0);
      |         S_AXI_AWPROT  : in  std_logic_vector(2 downto 0);
      |         S_AXI_AWVALID : in  std_logic;
      |         S_AXI_AWREADY : out std_logic;
      |         
      |         S_AXI_WLAST   : in  std_logic;
      |         S_AXI_WDATA   : in  std_logic_vector(C_S_AXI_DATA_WIDTH-1 downto 0);
      |         S_AXI_WSTRB   : in  std_logic_vector((C_S_AXI_DATA_WIDTH/8)-1 downto 0);
      |         S_AXI_WVALID  : in  std_logic;
      |         S_AXI_WREADY  : out std_logic;
      |         
      |         S_AXI_BRESP   : out std_logic_vector(1 downto 0);
      |         S_AXI_BID     : out std_logic_vector(C_S_AXI_ID_WIDTH-1 downto 0);
      |         S_AXI_BVALID  : out std_logic;
      |         S_AXI_BREADY  : in  std_logic;
      |         
      |         S_AXI_ARADDR  : in  std_logic_vector(C_S_AXI_ADDR_WIDTH-1 downto 0);
      |         S_AXI_ARID    : in  std_logic_vector(C_S_AXI_ID_WIDTH-1 downto 0);
      |         S_AXI_ARLEN   : in  std_logic_vector(C_S_AXI_ARLEN_WIDTH-1 downto 0);
      |         S_AXI_ARSIZE  : in  std_logic_vector(2 downto 0);
      |         S_AXI_ARBURST : in  std_logic_vector(1 downto 0);
      |         S_AXI_ARLOCK  : in  std_logic_vector(1 downto 0);
      |         S_AXI_ARCACHE : in  std_logic_vector(3 downto 0);
      |         S_AXI_ARPROT  : in  std_logic_vector(2 downto 0);
      |         S_AXI_ARVALID : in  std_logic;
      |         S_AXI_ARREADY : out std_logic;
      |         
      |         -- 'From Register'
      |         -- 'To Register'
      |         -- 'dac_en'
      |         sm_dac_en_dout : in std_logic_vector(1-1 downto 0);
      |         sm_dac_en_din  : out std_logic_vector(1-1 downto 0);
      |         sm_dac_en_en   : out std_logic;
      |         -- 'From FIFO'
      |         -- 'To FIFO'
      |         -- 'Shared Memory'
      | 
      |         S_AXI_RLAST   : out std_logic;
      |         S_AXI_RID     : out std_logic_vector(C_S_AXI_ID_WIDTH-1 downto 0);
      |         S_AXI_RDATA   : out std_logic_vector(C_S_AXI_DATA_WIDTH-1 downto 0);
      |         S_AXI_RRESP   : out std_logic_vector(1 downto 0);
      |         S_AXI_RVALID  : out std_logic;
      |         S_AXI_RREADY  : in  std_logic
      |     );
      | end entity axi_sgiface;
      | 
      | architecture IMP of axi_sgiface is
      | 
      | -- Internal signals for write channel.
      | signal S_AXI_BVALID_i       : std_logic;
      | signal S_AXI_BID_i          : std_logic_vector(C_S_AXI_ID_WIDTH-1 downto 0);
      | signal S_AXI_WREADY_i       : std_logic;
      |   
      | -- Internal signals for read channels.
      | signal S_AXI_ARLEN_i        : std_logic_vector(C_S_AXI_ARLEN_WIDTH-1 downto 0);
      | signal S_AXI_RLAST_i        : std_logic;
      | signal S_AXI_RREADY_i       : std_logic;
      | signal S_AXI_RVALID_i       : std_logic;
      | signal S_AXI_RDATA_i        : std_logic_vector(C_S_AXI_DATA_WIDTH-1 downto 0);
      | signal S_AXI_RID_i          : std_logic_vector(C_S_AXI_ID_WIDTH-1 downto 0);
      | 
      | -- for read channel
      | signal read_bank_addr_i     : std_logic_vector(C_S_AXI_BANK_ADDR_LEN-1 downto 0);
      | signal read_linear_addr_i   : std_logic_vector(C_S_AXI_LINEAR_ADDR_LEN-1 downto 0);
      | -- for write channel
      | signal write_bank_addr_i    : std_logic_vector(C_S_AXI_BANK_ADDR_LEN-1 downto 0);
      | signal write_linear_addr_i  : std_logic_vector(C_S_AXI_LINEAR_ADDR_LEN-1 downto 0);
      | 
      | signal reg_bank_out_i       : std_logic_vector(C_S_AXI_DATA_WIDTH-1 downto 0);
      | signal fifo_bank_out_i      : std_logic_vector(C_S_AXI_DATA_WIDTH-1 downto 0);
      | signal shmem_bank_out_i     : std_logic_vector(C_S_AXI_DATA_WIDTH-1 downto 0);
      |     
      | -- 'From Register'
      | -- 'To Register'
      | -- 'dac_en'
      | signal sm_dac_en_din_i   : std_logic_vector(C_S_AXI_DATA_WIDTH-1 downto 0);
      | signal sm_dac_en_en_i    : std_logic;
      | signal sm_dac_en_dout_i  : std_logic_vector(C_S_AXI_DATA_WIDTH-1 downto 0);
      | -- 'From FIFO'
      | -- 'To FIFO'
      | -- 'Shared Memory'
      | 
      | type t_read_state is (IDLE, READ_PREP, READ_DATA);
      | signal read_state : t_read_state;
      | 
      | type t_write_state is (IDLE, WRITE_DATA, WRITE_RESPONSE);
      | signal write_state : t_write_state;
      | 
      | type t_memmap_state is (READ, WRITE);
      | signal memmap_state : t_memmap_state;
      | 
      | constant C_READ_PREP_DELAY : std_logic_vector(1 downto 0) := "11";
      | 
      | signal read_prep_counter : std_logic_vector(1 downto 0);
      | signal read_addr_counter : std_logic_vector(C_S_AXI_ARLEN_WIDTH-1 downto 0);
      | signal read_data_counter : std_logic_vector(C_S_AXI_ARLEN_WIDTH-1 downto 0);
      | 
      | -- enable of shared BRAMs
      | signal s_shram_en : std_logic;
      | 
      | signal write_addr_valid : std_logic;
      | signal write_ready : std_logic;
      | 
      | -- 're' of From/To FIFOs
      | signal s_fifo_re : std_logic;
      | -- 'we' of To FIFOs
      | signal s_fifo_we : std_logic;
      | 
      | begin
      | 
      | -- enable for 'Shared Memory' blocks
      | 
      | -- conversion to match with the data bus width
      | -- 'From Register'
      | -- 'To Register'
      | -- 'dac_en'
      | sm_dac_en_din     <= sm_dac_en_din_i(1-1 downto 0);
      | sm_dac_en_en      <= sm_dac_en_en_i;
      | gen_sm_dac_en_dout_i: if (1 < C_S_AXI_DATA_WIDTH) generate
      |     sm_dac_en_dout_i(C_S_AXI_DATA_WIDTH-1 downto 1) <= (others => '0');
      | end generate gen_sm_dac_en_dout_i;
      | sm_dac_en_dout_i(1-1 downto 0) <= sm_dac_en_dout;
      | -- 'From FIFO'
      | -- 'To FIFO'
      | -- 'Shared Memory'
      | 
      | ReadWriteSelect: process(memmap_state) is begin
      |     if (memmap_state = READ) then
      |     else
      |     end if;
      | end process ReadWriteSelect;
      | 
      | -----------------------------------------------------------------------------
      | -- address for 'Shared Memory'
      | -----------------------------------------------------------------------------
      | SharedMemory_Addr_ResetN : process(AXI_AClk) is begin
      |     if (AXI_AClk'event and AXI_AClk = '1') then
      |         if (AXI_AResetN = '0') then
      |             memmap_state <= READ;
      |         else
      |             if (S_AXI_AWVALID = '1') then
      |                 -- write operation
      |                 memmap_state <= WRITE;
      |             elsif (S_AXI_ARVALID = '1') then
      |                 -- read operation
      |                 memmap_state <= READ;
      |             end if;
      |         end if;
      |     end if;
      | end process SharedMemory_Addr_ResetN;
      | 
      | -----------------------------------------------------------------------------
      | -- WRITE Command Control
      | -----------------------------------------------------------------------------
      | S_AXI_BID     <= S_AXI_BID_i;
      | S_AXI_BVALID  <= S_AXI_BVALID_i;
      | S_AXI_WREADY  <= S_AXI_WREADY_i;
      | -- No error checking
      | S_AXI_BRESP  <= (others=>'0');
      | 
      | PROC_AWREADY_ACK: process(read_state, write_state, S_AXI_ARVALID, S_AXI_AWVALID) is begin
      |     if (write_state = IDLE and S_AXI_AWVALID = '1' and read_state = IDLE) then
      |         S_AXI_AWREADY <= S_AXI_AWVALID;
      |     else
      |         S_AXI_AWREADY <= '0';
      |     end if;
      | end process PROC_AWREADY_ACK;
      | 
      | Cmd_Decode_Write: process(AXI_AClk) is begin
      |     if (AXI_AClk'event and AXI_AClk = '1') then
      |         if (AXI_AResetN = '0') then
      |             write_addr_valid    <= '0';
      |             write_ready         <= '0';
      |             s_fifo_we           <= '0';
      |             S_AXI_BVALID_i      <= '0';
      |             S_AXI_BID_i         <= (others => '0');
      |             write_bank_addr_i   <= (others => '0');
      |             write_linear_addr_i <= (others => '0');
      |         else
      |             if (write_state = IDLE) then
      |                 if (S_AXI_AWVALID = '1' and read_state = IDLE) then
      |                     -- reflect awid
      |                     S_AXI_BID_i <= S_AXI_AWID;
      | 
      |                     -- latch bank and linear addresses
      |                     write_bank_addr_i   <= S_AXI_AWADDR(C_S_AXI_TOTAL_ADDR_LEN-1 downto C_S_AXI_LINEAR_ADDR_LEN+2);
      |                     write_linear_addr_i <= S_AXI_AWADDR(C_S_AXI_LINEAR_ADDR_LEN+1 downto 2);
      |                     write_addr_valid <= '1';
      |                     s_fifo_we <= '1';
      | 
      |                     -- write state transition
      |                     write_state <= WRITE_DATA;
      |                 end if;
      |             elsif (write_state = WRITE_DATA) then
      |                 write_ready <= '1';
      |                 s_fifo_we <= '0';
      |                 write_addr_valid <= S_AXI_WVALID;
      |                 
      |                 if (S_AXI_WVALID = '1' and write_ready = '1') then
      |                     write_linear_addr_i <= Std_Logic_Vector(unsigned(write_linear_addr_i) + 1);
      |                 end if;
      | 
      |                 if (S_AXI_WLAST = '1' and write_ready = '1') then
      |                     -- start responding through B channel upon the last write data sample
      |                     S_AXI_BVALID_i <= '1';
      |                     -- write data is over
      |                     write_addr_valid <= '0';
      |                     write_ready <= '0';
      |                     -- write state transition
      |                     write_state <= WRITE_RESPONSE;
      |                 end if;
      |             elsif (write_state = WRITE_RESPONSE) then
      | 
      |                 if (S_AXI_BREADY = '1') then
      |                     -- write respond is over
      |                     S_AXI_BVALID_i <= '0';
      |                     S_AXI_BID_i <= (others => '0');
      | 
      |                     -- write state transition
      |                     write_state <= IDLE;
      |                 end if;
      |             end if;
      |         end if;
      |     end if;
      | end process Cmd_Decode_Write;
      | 
      | Write_Linear_Addr_Decode : process(AXI_AClk) is 
      | 
      | begin
      |     if (AXI_AClk'event and AXI_AClk = '1') then
      |         if (AXI_AResetN = '0') then
      |             -- 'To Register'
      |             -- dac_en din/en
      |             sm_dac_en_din_i <= (others => '0');
      |             sm_dac_en_en_i <= '0';
      |             -- 'To FIFO'
      |             -- 'Shared Memory'
      |         else
      |             -- default assignments
      | 
      |             -- 'To Register'
      |             if (unsigned(write_bank_addr_i) = 2) then
      |                 if (unsigned(write_linear_addr_i) = 0) then
      |                     -- dac_en din/en
      |                     sm_dac_en_din_i <= S_AXI_WDATA;
      |                     sm_dac_en_en_i  <= write_addr_valid;
      |                 end if;
      |             end if;        
      |         
      |         
      |         end if;
      |     end if;
      | end process Write_Linear_Addr_Decode;
      |  
      | -----------------------------------------------------------------------------
      | -- READ Control
      | -----------------------------------------------------------------------------
      | 
      | S_AXI_RDATA  <= S_AXI_RDATA_i;
      | S_AXI_RVALID  <= S_AXI_RVALID_i;
      | S_AXI_RLAST   <= S_AXI_RLAST_i;
      | S_AXI_RID     <= S_AXI_RID_i;
      | -- TODO: no error checking
      | S_AXI_RRESP <= (others=>'0');
      | 
      | PROC_ARREADY_ACK: process(read_state, S_AXI_ARVALID, write_state, S_AXI_AWVALID) is begin
      |     -- Note: WRITE has higher priority than READ
      |     if (read_state = IDLE and S_AXI_ARVALID = '1' and write_state = IDLE and S_AXI_AWVALID /= '1') then
      |         S_AXI_ARREADY <= S_AXI_ARVALID;
      |     else
      |         S_AXI_ARREADY <= '0';
      |     end if;
      | end process PROC_ARREADY_ACK;
      | 
      | S_AXI_WREADY_i <= write_ready;
      | 
      | Process_Sideband: process(write_state, read_state) is begin
      |     if (read_state = READ_PREP) then
      |         s_shram_en <= '1';
      |     elsif (read_state = READ_DATA) then
      |         s_shram_en <= S_AXI_RREADY;
      |     elsif (write_state = WRITE_DATA) then
      |         s_shram_en <= S_AXI_WVALID;
      |     else
      |         s_shram_en <= '0';
      |     end if;
      | end process Process_Sideband;
      | 
      | Cmd_Decode_Read: process(AXI_AClk) is begin
      |     if (AXI_AClk'event and AXI_AClk = '1') then
      |         if (AXI_AResetN = '0') then
      |             S_AXI_RVALID_i <= '0';
      |             read_bank_addr_i    <= (others => '0');
      |             read_linear_addr_i  <= (others => '0');
      |             S_AXI_ARLEN_i       <= (others => '0');
      |             S_AXI_RLAST_i       <= '0';
      |             S_AXI_RID_i         <= (others => '0');
      |             read_state          <= IDLE;
      |             read_prep_counter   <= (others => '0');
      |             read_addr_counter   <= (others => '0');
      |             read_data_counter   <= (others => '0');
      |         else
      |             -- default assignments
      |             s_fifo_re <= '0';
      | 
      |             if (read_state = IDLE) then
      |                 -- Note WRITE has higher priority than READ
      |                 if (S_AXI_ARVALID = '1' and write_state = IDLE and S_AXI_AWVALID /= '1') then
      |                     -- extract bank and linear addresses
      |                     read_bank_addr_i    <= S_AXI_ARADDR(C_S_AXI_TOTAL_ADDR_LEN-1 downto C_S_AXI_LINEAR_ADDR_LEN+2);
      |                     read_linear_addr_i  <= S_AXI_ARADDR(C_S_AXI_LINEAR_ADDR_LEN+1 downto 2);
      |                     s_fifo_re <= '1';
      | 
      |                     -- reflect arid
      |                     S_AXI_RID_i <= S_AXI_ARID;
      | 
      |                     -- load read liner address and data counter
      |                     read_addr_counter <= S_AXI_ARLEN;
      |                     read_data_counter <= S_AXI_ARLEN;
      | 
      |                     -- load read preparation counter
      |                     read_prep_counter <= C_READ_PREP_DELAY;
      |                     -- read state transition
      |                     read_state <= READ_PREP;
      |                 end if;
      |             elsif (read_state = READ_PREP) then
      |                 if (unsigned(read_prep_counter) = 0) then
      |                     if (unsigned(read_data_counter) = 0) then
      |                         -- tag the last data generated by the slave
      |                         S_AXI_RLAST_i <= '1';
      |                     end if;
      |                     -- valid data appears
      |                     S_AXI_RVALID_i <= '1';
      |                     -- read state transition
      |                     read_state <= READ_DATA;
      |                 else
      |                     -- decrease read preparation counter
      |                     read_prep_counter <= Std_Logic_Vector(unsigned(read_prep_counter) - 1);
      |                 end if;
      | 
      |                 if (unsigned(read_prep_counter) /= 3 and unsigned(read_addr_counter) /= 0) then
      |                     -- decrease address counter
      |                     read_addr_counter <= Std_Logic_Vector(unsigned(read_addr_counter) - 1);
      |                     -- increase linear address (no band crossing)
      |                     read_linear_addr_i <= Std_Logic_Vector(unsigned(read_linear_addr_i) + 1);
      |                 end if;
      |             elsif (read_state = READ_DATA) then
      |                 if (S_AXI_RREADY = '1') then
      |                     if (unsigned(read_data_counter) = 1) then
      |                         -- tag the last data generated by the slave
      |                         S_AXI_RLAST_i <= '1';
      |                     end if;
      | 
      |                     if (unsigned(read_data_counter) = 0) then
      |                         -- arid
      |                         S_AXI_RID_i <= (others => '0');
      |                         -- rlast
      |                         S_AXI_RLAST_i <= '0';
      |                         -- no more valid data
      |                         S_AXI_RVALID_i <= '0';
      |                         -- read state transition
      |                         read_state <= IDLE;
      |                     else
      |                         -- decrease read preparation counter
      |                         read_data_counter <= Std_Logic_Vector(unsigned(read_data_counter) - 1);
      | 
      |                         if (unsigned(read_addr_counter) /= 0) then
      |                             -- decrease address counter
      |                             read_addr_counter <= Std_Logic_Vector(unsigned(read_addr_counter) - 1);
      |                             -- increase linear address (no band crossing)
      |                             read_linear_addr_i <= Std_Logic_Vector(unsigned(read_linear_addr_i) + 1);
      |                         end if;
      |                     end if;
      |                 end if;
      |             end if;
      | 
      |         end if;
      |     end if;
      | end process Cmd_Decode_Read;
      | 
      | Read_Linear_Addr_Decode : process(AXI_AClk) is begin
      |     if (AXI_AClk'event and AXI_AClk = '1') then
      |         if (AXI_AResetN = '0') then
      |             reg_bank_out_i   <= (others => '0');
      |             fifo_bank_out_i  <= (others => '0');
      |             shmem_bank_out_i <= (others => '0');
      |             S_AXI_RDATA_i    <= (others => '0');
      |         else
      |             if (unsigned(read_bank_addr_i) = 2) then
      |                 -- 'From Register'
      | 
      |                 S_AXI_RDATA_i <= reg_bank_out_i;
      |             elsif (unsigned(read_bank_addr_i) = 1) then
      |                 -- 'From FIFO'
      |                 -- 'To FIFO'
      | 
      |                 S_AXI_RDATA_i <= fifo_bank_out_i;
      |             elsif (unsigned(read_bank_addr_i) = 0 and s_shram_en = '1') then
      |                 -- 'Shared Memory'
      | 
      |                 S_AXI_RDATA_i <= shmem_bank_out_i;
      |             end if;
      |         end if;
      |     end if;
      | end process Read_Linear_Addr_Decode;
      | 
      | end architecture IMP;
      settings: infoedit=For use with EDK Processor block.
  wires:
  memmap/13 -> To Register/2
  memmap/12 -> To Register/1
  memmap/11 -> S_AXI_WREADY/1
  memmap/10 -> S_AXI_RVALID/1
  memmap/9 -> S_AXI_RRESP/1
  memmap/8 -> S_AXI_RLAST/1
  memmap/7 -> S_AXI_RID/1
  memmap/6 -> S_AXI_RDATA/1
  memmap/5 -> S_AXI_BVALID/1
  memmap/4 -> S_AXI_BRESP/1
  memmap/3 -> S_AXI_BID/1
  memmap/2 -> S_AXI_AWREADY/1
  memmap/1 -> S_AXI_ARREADY/1
  S_AXI_WVALID/1 -> memmap/25
  S_AXI_WSTRB/1 -> memmap/24
  S_AXI_WLAST/1 -> memmap/23
  S_AXI_WDATA/1 -> memmap/22
  S_AXI_RREADY/1 -> memmap/21
  S_AXI_BREADY/1 -> memmap/20
  S_AXI_AWVALID/1 -> memmap/19
  S_AXI_AWSIZE/1 -> memmap/18
  S_AXI_AWPROT/1 -> memmap/17
  S_AXI_AWLOCK/1 -> memmap/16
  S_AXI_AWLEN/1 -> memmap/15
  S_AXI_AWID/1 -> memmap/14
  S_AXI_AWCACHE/1 -> memmap/13
  S_AXI_AWBURST/1 -> memmap/12
  S_AXI_AWADDR/1 -> memmap/11
  S_AXI_ARVALID/1 -> memmap/10
  S_AXI_ARSIZE/1 -> memmap/9
  S_AXI_ARPROT/1 -> memmap/8
  S_AXI_ARLOCK/1 -> memmap/7
  S_AXI_ARLEN/1 -> memmap/6
  S_AXI_ARID/1 -> memmap/5
  S_AXI_ARCACHE/1 -> memmap/4
  S_AXI_ARBURST/1 -> memmap/3
  S_AXI_ARADDR/1 -> memmap/2
  AXI_ARESETN/1 -> memmap/1
  To Register/1 -> memmap/26
  S_AXI_WREADY/1 -> Terminator10/1
  S_AXI_RVALID/1 -> Terminator9/1
  S_AXI_RRESP/1 -> Terminator8/1
  S_AXI_RLAST/1 -> Terminator7/1
  S_AXI_RID/1 -> Terminator6/1
  S_AXI_RDATA/1 -> Terminator5/1
  S_AXI_BVALID/1 -> Terminator4/1
  S_AXI_BRESP/1 -> Terminator3/1
  S_AXI_BID/1 -> Terminator2/1
  S_AXI_AWREADY/1 -> Terminator1/1
  S_AXI_ARREADY/1 -> Terminator/1
  Constant24/1 -> S_AXI_WVALID/1
  Constant23/1 -> S_AXI_WSTRB/1
  Constant22/1 -> S_AXI_WLAST/1
  Constant21/1 -> S_AXI_WDATA/1
  Constant20/1 -> S_AXI_RREADY/1
  Constant19/1 -> S_AXI_BREADY/1
  Constant18/1 -> S_AXI_AWVALID/1
  Constant17/1 -> S_AXI_AWSIZE/1
  Constant16/1 -> S_AXI_AWPROT/1
  Constant15/1 -> S_AXI_AWLOCK/1
  Constant14/1 -> S_AXI_AWLEN/1
  Constant13/1 -> S_AXI_AWID/1
  Constant12/1 -> S_AXI_AWCACHE/1
  Constant11/1 -> S_AXI_AWBURST/1
  Constant10/1 -> S_AXI_AWADDR/1
  Constant9/1 -> S_AXI_ARVALID/1
  Constant8/1 -> S_AXI_ARSIZE/1
  Constant7/1 -> S_AXI_ARPROT/1
  Constant6/1 -> S_AXI_ARLOCK/1
  Constant5/1 -> S_AXI_ARLEN/1
  Constant4/1 -> S_AXI_ARID/1
  Constant3/1 -> S_AXI_ARCACHE/1
  Constant2/1 -> S_AXI_ARBURST/1
  Constant1/1 -> S_AXI_ARADDR/1
  Constant/1 -> AXI_ARESETN/1
